simulink model "CodeGen_subsystem0"  (R2023b)
settings: Solver=FixedStepDiscrete  StartTime=0.0  StopTime=20  FixedStep=0.01  MaxStep=0.01  RelTol=1e-3  EnableMultiTasking=on
model workspace (MAT data in the model file):
  Diff_i = Simulink.Parameter
  Diff_i.Value = [1; 1; 1; 1]
  Diff_i.DataType = 'auto'
  Diff_i.Complexity = 'real'
  Diff_i.Dimensions = [4 1]
  Get_i = Simulink.Parameter
  Get_i.Value = [17; 16; 16; 17]
  Get_i.DataType = 'auto'
  Get_i.Complexity = 'real'
  Get_i.Dimensions = [4 1]
  Off_i = Simulink.Parameter
  Off_i.Value = [20; 20; 20; 20]
  Off_i.DataType = 'auto'
  Off_i.Complexity = 'real'
  Off_i.Dimensions = [4 1]
  On_i = Simulink.Parameter
  On_i.Value = [19; 19; 19; 19]
  On_i.DataType = 'auto'
  On_i.Complexity = 'real'
  On_i.Dimensions = [4 1]
settings Model: ExtModeTrigDuration=2  Creator=Asus  LastModifiedBy=Asus
settings DataIOCC: SaveOutput=off  SaveTime=off
settings OptimizationCC: EnhancedBackFolding=on  PassReuseOutputArgsAs=Individual arguments  ZeroExternalMemoryAtStartup=off  ZeroInternalMemoryAtStartup=off  MaxStackSize=64  OptimizeBlockOrder=speed  DifferentSizesBufferReuse=on  OptimizationCustomize=off  EfficientTunableParamExpr=on
settings DebuggingCC: ParameterTunabilityLossMsg=error
settings HardwareCC: ProdBitPerInt=16  ProdBitPerPointer=16  ProdBitPerSizeT=16  ProdBitPerPtrDiffT=16  ProdLargestAtomicFloat=None  ProdWordSize=8  ProdHWDeviceType=Atmel->AVR
settings SFSimCC: MATLABDynamicMemAlloc=off
settings RTWCC: Description=Embedded Coder  SystemTargetFile=ert.tlc  HardwareBoard=Arduino Uno  GenCodeOnly=on  TemplateMakefile=ert_default_tmf  Toolchain=Arduino AVR  BuildConfiguration=Faster Runs
settings CodeAppCC: ForceParamTrailComments=on  IgnoreCustomStorageClasses=off  OperatorAnnotations=on  SimulinkDataObjDesc=on  SFDataObjDesc=on  InsertBlockDesc=on
settings ERTTargetCC: SupportContinuousTime=on  SupportVariableSizeSignals=on  ExtModeTransport=3  ExtModeStaticAlloc=on  ExtModeAutomaticAllocSize=off  ExtModeStaticAllocSize=250  ExtModeMexFile=ext_xcp  ExtModeIntrfLevel=Level2 - Open

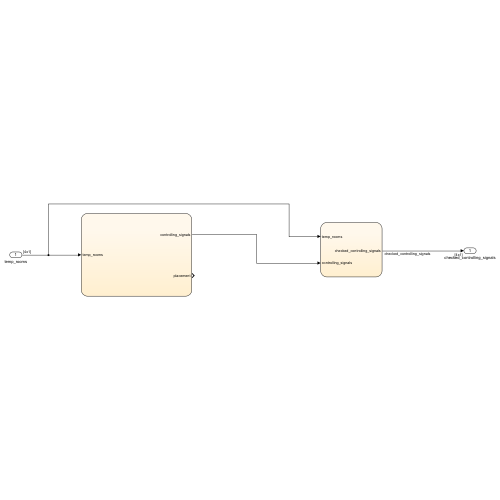
[thumbnail: Simulink's stored preview of the top-level diagram]
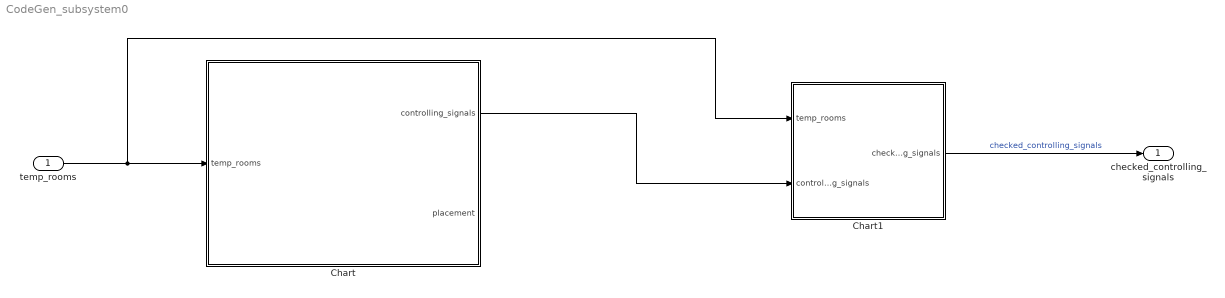
== system CodeGen_subsystem0 ==
  temp_rooms : Inport  RequirementInfo={} %GIDa_89e873dc_ec86_4052_adc9_6d25efaf2334  OutDataTypeStr=double  PortDimensions=[4 1]
  Chart : Stateflow chart  RequirementInfo={} %GIDa_792f3f4d_6d0b_4891_85c1_c577bb1f452b  TreatAsAtomicUnit=on
  Chart1 : Stateflow chart  RequirementInfo={} %GIDa_f6153acd_8b95_4da1_9ac2_0d86a288dd79  TreatAsAtomicUnit=on
  checked_controlling_signals : Outport  RequirementInfo={} %GIDa_60651ffb_267d_4416_b72e_17cccdcfedcd  OutDataTypeStr=double  PortDimensions=[4 1]  SampleTime=[0,1]
  wires:
  temp_rooms/1 -> Chart/1(temp_rooms), Chart1/1(temp_rooms)
  Chart/1(controlling_signals) -> Chart1/2(controlling_signals)
  Chart1/1(checked_controlling_signals) -> checked_controlling_signals/1  "checked_controlling_signals"

== stateflow chart CodeGen_subsystem0/Chart ==
  state two_three
    during:
    placement = 23;
    if(temp_rooms(2) <= On_i(2))
    controlling_signals(2) = 1;
    end
    if(temp_rooms(3) <= On_i(3))
    controlling_signals(3) = 1;
    end
    if(temp_rooms(2) >= Off_i(2))
    controlling_signals(2) = 0;
    end
    if(temp_rooms(3) >= Off_i(3))
    controlling_signals(3) = 0;
    end
    exit:
    controlling_signals(:) = 0;
  state one_two
    during:
    placement = 12;
    if(temp_rooms(1) <= On_i(1))
    controlling_signals(1) = 1;
    end
    if(temp_rooms(2) <= On_i(2))
    controlling_signals(2) = 1;
    end
    if(temp_rooms(1) >= Off_i(1))
    controlling_signals(1) = 0;
    end
    if(temp_rooms(2) >= Off_i(2))
    controlling_signals(3) = 0;
    end
    exit:
    controlling_signals(:) = 0;
  state one_three
    during:
    placement = 13
    if(temp_rooms(1) <= On_i(1))
    controlling_signals(1) = 1;
    end
    if(temp_rooms(3) <= On_i(3))
    controlling_signals(3) = 1;
    end
    if(temp_rooms(1) >= Off_i(1))
    controlling_signals(1) = 0;
    end
    if(temp_rooms(3) >= Off_i(3))
    controlling_signals(3) = 0;
    end
    exit:
    controlling_signals(:) = 0;
  state one_four
    during:
    placement = 14;
    if(temp_rooms(1) <= On_i(1))
    controlling_signals(1) = 1;
    end
    if(temp_rooms(4) <= On_i(4))
    controlling_signals(4) = 1;
    end
    if(temp_rooms(1) >= Off_i(1))
    controlling_signals(1) = 0;
    end
    if(temp_rooms(4) >= Off_i(4))
    controlling_signals(4) = 0;
    end
    exit:
    controlling_signals(:) = 0;
  state two_four
    during:
    placement = 24;
    if(temp_rooms(2) <= On_i(2))
    controlling_signals(2) = 1;
    end
    if(temp_rooms(4) <= On_i(4))
    controlling_signals(4) = 1;
    end
    if(temp_rooms(2) >= Off_i(2))
    controlling_signals(2) = 0;
    end
    if(temp_rooms(4) >= Off_i(4))
    controlling_signals(4) = 0;
    end
    exit:
    controlling_signals(:) = 0;
  state three_four
    during:
    placement = 34;
    if(temp_rooms(3) <= On_i(3))
    controlling_signals(3) = 1;
    end
    if(temp_rooms(4) <= On_i(4))
    controlling_signals(4) = 1;
    end
    if(temp_rooms(3) >= Off_i(3))
    controlling_signals(3) = 0;
    end
    if(temp_rooms(4) >= Off_i(4))
    controlling_signals(4) = 0;
    end
    exit:
    controlling_signals(:) = 0;
  one_three -> two_three [order 3] : [temp_rooms(1) - temp_rooms(2) >= Diff_i(2) && temp_rooms(2) <= Get_i(2)]
  two_three -> one_three [order 3] : [temp_rooms(2) - temp_rooms(1) >= Diff_i(1) && temp_rooms(1) <= Get_i(1)]
  one_three -> one_four [order 2] : [temp_rooms(3) - temp_rooms(4) >= Diff_i(4) && temp_rooms(4) <= Get_i(4)]
  (default) -> two_three
  one_two -> one_three [order 3] : [temp_rooms(2) - temp_rooms(3) >= Diff_i(3) && temp_rooms(3) <= Get_i(3)]
  two_three -> one_two [order 1] : [temp_rooms(3) - temp_rooms(1) >= Diff_i(1) && temp_rooms(1) <= Get_i(1)]
  one_three -> one_two [order 1] : [temp_rooms(3) - temp_rooms(2) >= Diff_i(2) && temp_rooms(2) <= Get_i(2)]
  one_two -> two_three [order 1] : [temp_rooms(1) - temp_rooms(3) >= Diff_i(3) && temp_rooms(3) <= Get_i(3)]
  one_two -> one_four [order 4] : [temp_rooms(2) - temp_rooms(4) >= Diff_i(4) && temp_rooms(4) <= Get_i(4)]
  three_four -> two_three [order 3] : [temp_rooms(4) - temp_rooms(2) >= Diff_i(2) && temp_rooms(2) <= Get_i(2)]
  two_four -> two_three [order 4] : [temp_rooms(4) - temp_rooms(3) >= Diff_i(3) && temp_rooms(3) <= Get_i(3)]
  two_three -> three_four [order 4] : [temp_rooms(2) - temp_rooms(4) >= Diff_i(4) && temp_rooms(4) <= Get_i(4)]
  two_three -> two_four [order 2] : [temp_rooms(3) - temp_rooms(4) >= Diff_i(4) && temp_rooms(4) <= Get_i(4)]
  one_four -> one_two [order 3] : [temp_rooms(4) - temp_rooms(2) >= Diff_i(2) && temp_rooms(2) <= Get_i(2)]
  one_four -> one_three [order 4] : [temp_rooms(4) - temp_rooms(3) >= Diff_i(3) && temp_rooms(3) <= Get_i(3)]
  one_two -> two_four [order 2] : [temp_rooms(1) - temp_rooms(4) >= Diff_i(4) && temp_rooms(4) <= Get_i(4)]
  two_four -> one_two [order 3] : [temp_rooms(4) - temp_rooms(1) >= Diff_i(1) && temp_rooms(1) <= Get_i(1)]
  one_three -> three_four [order 4] : [temp_rooms(3) - temp_rooms(1) >= Diff_i(1) && temp_rooms(1) <= Get_i(1)]
  three_four -> one_three [order 4] : [temp_rooms(4) - temp_rooms(1) >= Diff_i(1) && temp_rooms(1) <= Get_i(1)]
  one_four -> two_four [order 1] : [temp_rooms(1) - temp_rooms(2) >= Diff_i(2) && temp_rooms(2) <= Get_i(2)]
  two_four -> three_four [order 2] : [temp_rooms(2) - temp_rooms(3) >= Diff_i(3) && temp_rooms(3) <= Get_i(3)]
  three_four -> two_four [order 1] : [temp_rooms(3) - temp_rooms(2) >= Diff_i(2) && temp_rooms(2) <= Get_i(2)]
  two_four -> one_four [order 1] : [temp_rooms(2) - temp_rooms(1) >= Diff_i(1) && temp_rooms(1) <= Get_i(1)]
  three_four -> one_four [order 2] : [temp_rooms(3) - temp_rooms(1) >= Diff_i(1) && temp_rooms(1) <= Get_i(1)]
  one_four -> three_four [order 2] : [temp_rooms(1) - temp_rooms(3) >= Diff_i(3) && temp_rooms(3) <= Get_i(3)]
  data: On_i parameter; Off_i parameter; Get_i parameter; Diff_i parameter; temp_rooms input size=[4 1]; controlling_signals output =[0; 0; 0; 0]; placement output

== stateflow chart CodeGen_subsystem0/Chart1 ==
  state safe
    during:
    checked_controlling_signals = controlling_signals
  state unsafe_sum
  (default) -> safe
  safe -> unsafe_sum : [sum(controlling_signals) > 2 || (controlling_signals(1) == 1 && temp_rooms(1) > Off_i(1)) || (controlling_signals(2) == 1 && temp_rooms(2) > Off_i(2)) || (controlling_signals(3) == 1 && temp_rooms(3) > Off_i(3)) || (controlling_signals(4) == 1 && temp_rooms(4) > Off_i(4))]{checked_controlling_signals(:) = 0}
  unsafe_sum -> safe : [~(sum(controlling_signals) > 2 || (controlling_signals(1) == 1 && temp_rooms(1) > Off_i(1)) || (controlling_signals(2) == 1 && temp_rooms(2) > Off_i(2)) || (controlling_signals(3) == 1 && temp_rooms(3) > Off_i(3)) || (controlling_signals(4) == 1 && temp_rooms(4) > Off_i(4)))]
  data: On_i parameter; Off_i parameter; temp_rooms input; controlling_signals input; checked_controlling_signals output =[0; 0; 0; 0]
